simulink model "a3_4_example_trigonometry"  (R2018a)
settings: Solver=VariableStepAuto  StartTime=0.0  StopTime=10.0  RelTol=1e-3
settings Model: Creator=r0x6f736f646f  LastModifiedBy=r0x6f736f646f

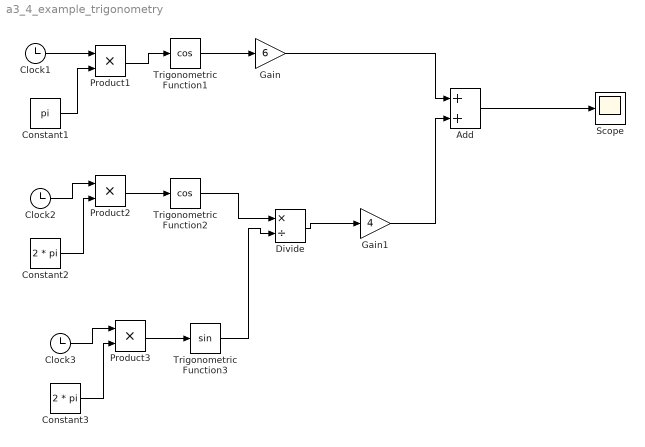
== system a3_4_example_trigonometry ==
  Add : Sum
  Clock1 : Clock
  Clock2 : Clock
  Clock3 : Clock
  Constant1 : Constant  Value=pi
  Constant2 : Constant  Value=2 * pi
  Constant3 : Constant  Value=2 * pi
  Divide : Product  Inputs=*/
  Gain : Gain  Gain=6
  Gain1 : Gain  Gain=4
  Product1 : Product
  Product2 : Product
  Product3 : Product
  Scope : Scope
  Trigonometric Function1 : Trigonometry  Operator=cos
  Trigonometric Function2 : Trigonometry  Operator=cos
  Trigonometric Function3 : Trigonometry
  wires:
  Clock1/1 -> Product1/1
  Constant1/1 -> Product1/2
  Product1/1 -> Trigonometric Function1/1
  Trigonometric Function1/1 -> Gain/1
  Clock2/1 -> Product2/1
  Constant2/1 -> Product2/2
  Trigonometric Function2/1 -> Divide/1
  Product2/1 -> Trigonometric Function2/1
  Trigonometric Function3/1 -> Divide/2
  Clock3/1 -> Product3/1
  Product3/1 -> Trigonometric Function3/1
  Constant3/1 -> Product3/2
  Divide/1 -> Gain1/1
  Gain/1 -> Add/1
  Gain1/1 -> Add/2
  Add/1 -> Scope/1
